simulink model "IMU_test"  (R2014b)
settings: Solver=FixedStepDiscrete  SolverMode=SingleTasking  StartTime=0.0  StopTime=inf  RelTol=1e-3
libraries: BeagleBoneBlackCom x1
settings Model: SimulationMode=external  Creator=Sebastian  LastModifiedBy=Sebastian
settings OptimizationCC: OptimizeModelRefInitCode=on  LifeSpan=1  MaxStackSize=64
settings DebuggingCC: UnderspecifiedInitializationDetection=Classic  MergeDetectMultiDrivingBlocksExec=none
settings HardwareCC: ProdLargestAtomicInteger=Long  ProdLargestAtomicFloat=Double  ProdEndianess=LittleEndian  ProdHWDeviceType=ARM Compatible->ARM Cortex
settings RTWCC: SystemTargetFile=ert.tlc  TLCOptions=-aInlineSetEventsForThisBaseRateFcn=TLC_FALSE -aSuppressMultiTaskScheduler=TLC_FALSE  TemplateMakefile=ert_default_tmf  Description=Embedded Coder  GenerateReport=on  RTWVerbose=off  ProcessScript=ert_make_rtw_hook  Toolchain=Linaro Toolchain v4.8  IncludeHyperlinkInReport=on  LaunchReport=on
settings CodeAppCC: IgnoreCustomStorageClasses=off
settings ERTTargetCC: SupportNonInlinedSFcns=on

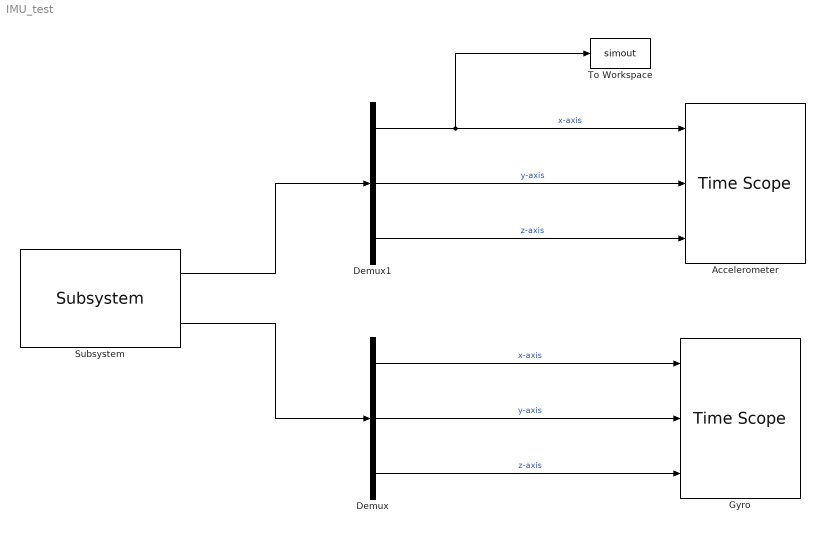
== system IMU_test ==
  Accelerometer : TimeScope  DefaultConfigurationName=spbscopes.TimeScopeBlockCfg  NumInputPorts=3
  Demux : Demux  Outputs=3
  Demux1 : Demux  Outputs=3
  Gyro : TimeScope  DefaultConfigurationName=spbscopes.TimeScopeBlockCfg  NumInputPorts=3
  Subsystem : BeagleBoneBlackCom/Subsystem  accSens=2 g  gyroSens=1000 degree/s
  To Workspace : ToWorkspace  VariableName=simout  SaveFormat=Structure With Time  SampleTime=-1
  wires:
  Demux/1 -> Gyro/1  "x-axis"
  Demux/2 -> Gyro/2  "y-axis"
  Demux1/1 -> Accelerometer/1, To Workspace/1  "x-axis"
  Demux1/2 -> Accelerometer/2  "y-axis"
  Demux1/3 -> Accelerometer/3  "z-axis"
  Subsystem/1 -> Demux1/1
  Subsystem/2 -> Demux/1
  Demux/3 -> Gyro/3  "z-axis"
